simulink model "three_phase_inverter_LCL"  (R2024a)
settings: Solver=VariableStepAuto  StartTime=0.0  StopTime=10.0  RelTol=1e-3
libraries: spsSeriesRLCBranchLib x12, simulink x7, spsIGBTLib x6, slpidlib x4, spsabctodq0Lib x3, spsGroundLib x2, spsSawtoothGeneratorLib x2, spsTHDLib x2, spsDCVoltageSourceLib x1, spsThreePhaseParallelRLCBranchLib x1, spsThreePhaseVIMeasurementLib x1, sps_lib x1
settings Model: Creator=rizzilouise  LastModifiedBy=rizzilouise
settings SolverCC: ZeroCrossAlgorithm=Adaptive
settings DebuggingCC: MaskedZcDiagnostic=none  IgnoredZcDiagnostic=none  InitInArrayFormatMsg=none

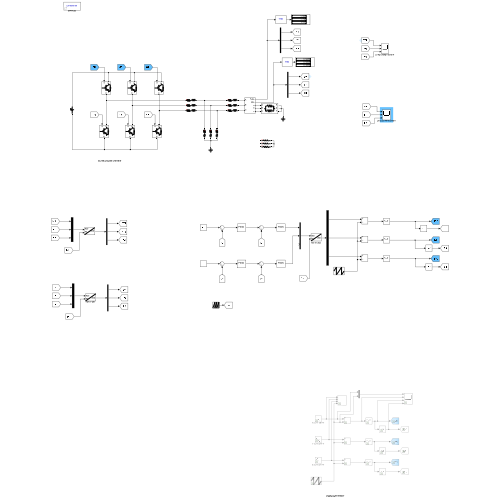
[thumbnail: Simulink's stored preview of the top-level diagram]
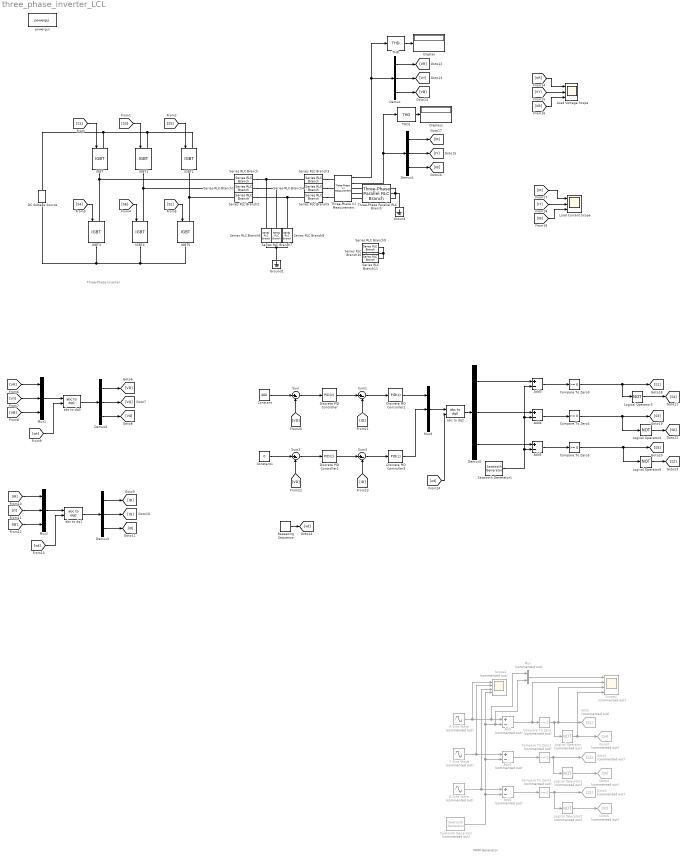
== system three_phase_inverter_LCL ==
  note: PWM Generator
  note: Three-Phase Inverter
  Add : Sum  Commented=on  Inputs=+-
  Add1 : Sum  Commented=on  Inputs=+-
  Add2 : Sum  Commented=on  Inputs=+-
  Add3 : Sum  Inputs=+-
  Add4 : Sum  Inputs=+-
  Add5 : Sum  Inputs=+-
  B Sine Wave : Sin  Commented=on  Frequency=2*pi*50  Phase=-2*pi/3  SampleTime=0
  Compare To Zero : simulink/Logic and Bit Operations/Compare To Zero  Commented=on  relop=>=  OutDataTypeStr=boolean
  Compare To Zero1 : simulink/Logic and Bit Operations/Compare To Zero  Commented=on  relop=>=  OutDataTypeStr=boolean
  Compare To Zero2 : simulink/Logic and Bit Operations/Compare To Zero  Commented=on  relop=>=  OutDataTypeStr=boolean
  Compare To Zero3 : simulink/Logic and Bit Operations/Compare To Zero  relop=>=  OutDataTypeStr=boolean
  Compare To Zero4 : simulink/Logic and Bit Operations/Compare To Zero  relop=>=  OutDataTypeStr=boolean
  Compare To Zero5 : simulink/Logic and Bit Operations/Compare To Zero  relop=>=  OutDataTypeStr=boolean
  Constant : Constant  Value=400
  Constant1 : Constant  Value=0
  DC Voltage Source : spsDCVoltageSourceLib/DC Voltage Source  Amplitude=230  Measurements=None
  Demux{,1..4} (5 alike) : Demux  Outputs=3
  Discrete PID Controller{,1..3} (4 alike) : slpidlib/PID Controller  Controller=PID  Form=Parallel  TimeDomain=Discrete-time  UseExternalTs=off  SampleTime=-1  IntegratorMethod=Forward Euler  FilterMethod=Forward Euler  ControllerParametersSource=internal  P=1  I=1  UseKiTs=off  D=0  UseExternalDerivativeSource=off  N=100  UseFilter=on  TunerSelectOption=Transfer Function Based (PID Tuner App)  InitialConditionSource=internal  InitialConditionForIntegrator=0  InitialConditionForFilter=0  DifferentiatorICPrevScaledInput=0  ExternalReset=none  TrackingMode=off  Kt=1  LimitOutput=off  SatLimitsSource=internal  UpperSaturationLimit=inf  LowerSaturationLimit=-inf  LinearizeAsGain=off  AntiWindupMode=none  Kb=1  LimitIntegrator=off  UpperIntegratorSaturationLimit=inf  LowerIntegratorSaturationLimit=-inf  POutMin=[]  POutMax=[]  IOutMin=[]  IOutMax=[]  DOutMin=[]  DOutMax=[]  NOutMin=[]  NOutMax=[]  SumOutMin=[]  SumOutMax=[]  SaturationOutMin=[]  SaturationOutMax=[]  PParamMin=[]  PParamMax=[]  IParamMin=[]  IParamMax=[]  DParamMin=[]  DParamMax=[]  NParamMin=[]  NParamMax=[]  KbParamMin=[]  KbParamMax=[]  KtParamMin=[]  KtParamMax=[]  KbOutMin=[]  KbOutMax=[]  KtOutMin=[]  KtOutMax=[]  IntegratorOutMin=[]  IntegratorOutMax=[]  FilterOutMin=[]  FilterOutMax=[]  SumI1OutMin=[]  SumI1OutMax=[]  SumI2OutMin=[]  SumI2OutMax=[]  SumI3OutMin=[]  SumI3OutMax=[]  SumI4OutMin=[]  SumI4OutMax=[]  SumDOutMin=[]  SumDOutMax=[]  DifferentiatorOutMin=[]  DifferentiatorOutMax=[]  FilterDiffOutCoefMin=[]  FilterDiffOutCoefMax=[]  ReciprocalOutMin=[]  ReciprocalOutMax=[]  SumDenOutMin=[]  SumDenOutMax=[]  SumNumOutMin=[]  SumNumOutMax=[]  DivideOutMin=[]  DivideOutMax=[]  UdiffTsProdOutMin=[]  UdiffTsProdOutMax=[]  NTsProdOutMin=[]  NTsProdOutMax=[]  UintegralTsProdOutMin=[]  UintegralTsProdOutMax=[]  UngainTsProdOutMin=[]  UngainTsProdOutMax=[]  ClampingZeroOutDataTypeStr=Inherit: Inherit via back propagation  ClampingZeroOutMin=[]  ClampingZeroOutMax=[]  FilterDenConstantOutDataTypeStr=Inherit: Inherit via back propagation  FilterDenConstantOutMin=[]  FilterDenConstantOutMax=[]  PCopyOutDataTypeStr=Inherit: Inherit via back propagation  PCopyOutMin=[]  PCopyOutMax=[]  NCopyOutDataTypeStr=Inherit: Inherit via back propagation  NCopyOutMin=[]  NCopyOutMax=[]  IntegratorContinuousStateAttributes=''  IntegratorStateMustResolveToSignalObject=off  IntegratorRTWStateStorageClass=Auto  FilterContinuousStateAttributes=''  FilterStateMustResolveToSignalObject=off  FilterRTWStateStorageClass=Auto  ParallelPVariant=InternalParameters  IdealPVariant=Disabled  IVariant=InternalParameters  DVariant=InternalParameters  IntegratorVariant=Discrete  SatVariant=Disabled  AWVariant=Passthrough  PCopyVariant=Disabled  TRVariant=Disabled  FdbkBlocksVariant=Forward  IdealPFdbkVariant=Disabled  SatFdbkVariant=Disabled  DerivativeFilterVariant=ForwardEulerFilter  NVariant=InternalParameters  NCopyVariant=Disabled  FilterICVariant=InternalICsFilter  IntegratorICVariant=InternalICs  ExternalResetVariant=Disabled  TRSumVariant=Passthrough  SumFdbkVariant=Disabled  SumVariant=Sum_PID  TsampFilterVariant=InternalTs  TsampNgainVariant=Passthrough  TsampIntegralVariant=Disabled_SignalSpec  ExternalSaturationOutDataTypeStr=Inherit: Same as second input  DerivativeSourceVariant=ErrorSignal
      settings: LibrarySourceBlock=simulink/Discrete/Discrete PID Controller
  Display : Display
  Display1 : Display
  Goto : Goto  Commented=on  GotoTag=S1
  Goto1 : Goto  Commented=on  GotoTag=S3
  Goto2 : Goto  Commented=on  GotoTag=S5
  Goto3 : Goto  Commented=on  GotoTag=S4
  Goto4 : Goto  Commented=on  GotoTag=S6
  Goto5 : Goto  Commented=on  GotoTag=S2
  Ground : spsGroundLib/Ground  LConnTagsString=a
  Ground1 : spsGroundLib/Ground  LConnTagsString=a
  IGBT{,1..5} (6 alike) : spsIGBTLib/IGBT  Ron=0.001  Lon=0  Vf=1  Tf=1e-6  Tt=2e-6  IC=0  Rs=1e5  Cs=inf  Measurements=off
  Load Current Scope : Scope  NumInputPorts=3
  Load Voltage Scope : Scope  NumInputPorts=3
  Logical Operator : Logic  Commented=on  Operator=NOT  AllPortsSameDT=off  OutDataTypeStr=boolean
  Logical Operator1 : Logic  Commented=on  Operator=NOT  AllPortsSameDT=off  OutDataTypeStr=boolean
  Logical Operator2 : Logic  Commented=on  Operator=NOT  AllPortsSameDT=off  OutDataTypeStr=boolean
  Logical Operator3 : Logic  Operator=NOT  AllPortsSameDT=off  OutDataTypeStr=boolean
  Logical Operator4 : Logic  Operator=NOT  AllPortsSameDT=off  OutDataTypeStr=boolean
  Logical Operator5 : Logic  Operator=NOT  AllPortsSameDT=off  OutDataTypeStr=boolean
  Mux : Mux  Commented=on  Inputs=2
  Mux1 : Mux  Inputs=3
  Mux2 : Mux  Inputs=3
  Mux3 : Mux  Inputs=3
  R Sine Wave : Sin  Commented=on  Frequency=2*pi*50  SampleTime=0
  Repeating Sequence : simulink/Sources/Repeating Sequence  rep_seq_t=[0 20e-3]  rep_seq_y=[0 2*pi]
  Sawtooth Generator : spsSawtoothGeneratorLib/Sawtooth Generator  Commented=on  Freq=10e3  Phase=180  Ts=0
  Sawtooth Generator1 : spsSawtoothGeneratorLib/Sawtooth Generator  Freq=10e3  Phase=180  Ts=0
  Scope1 : Scope  Commented=on  NumInputPorts=4
  Scope2 : Scope  Commented=on  NumInputPorts=4
  Series RLC Branch{,1..5} (6 alike) : spsSeriesRLCBranchLib/Series RLC Branch  LConnTagsString=__new0  RConnTagsString=__new0  BranchType=RL  Resistance=20e-3  Inductance=500e-6  SetiL0=off  InitialCurrent=0  Capacitance=1e-6  Setx0=off  InitialVoltage=0  Measurements=None
  Series RLC Branch10 : spsSeriesRLCBranchLib/Series RLC Branch  LConnTagsString=__new0  RConnTagsString=__new0  BranchType=R  Resistance=1.1  Inductance=1e-3  SetiL0=off  InitialCurrent=0  Capacitance=1e-6  Setx0=off  InitialVoltage=0  Measurements=None
  Series RLC Branch11 : spsSeriesRLCBranchLib/Series RLC Branch  LConnTagsString=__new0  RConnTagsString=__new0  BranchType=R  Resistance=1.1  Inductance=1e-3  SetiL0=off  InitialCurrent=0  Capacitance=1e-6  Setx0=off  InitialVoltage=0  Measurements=None
  Series RLC Branch6 : spsSeriesRLCBranchLib/Series RLC Branch  LConnTagsString=__new0  RConnTagsString=__new0  BranchType=RC  Resistance=20e-3  Inductance=1e-3  SetiL0=off  InitialCurrent=0  Capacitance=100e-6  Setx0=off  InitialVoltage=0  Measurements=None
  Series RLC Branch7 : spsSeriesRLCBranchLib/Series RLC Branch  LConnTagsString=__new0  RConnTagsString=__new0  BranchType=RC  Resistance=20e-3  Inductance=1e-3  SetiL0=off  InitialCurrent=0  Capacitance=100e-6  Setx0=off  InitialVoltage=0  Measurements=None
  Series RLC Branch8 : spsSeriesRLCBranchLib/Series RLC Branch  LConnTagsString=__new0  RConnTagsString=__new0  BranchType=RC  Resistance=20e-3  Inductance=1e-3  SetiL0=off  InitialCurrent=0  Capacitance=100e-6  Setx0=off  InitialVoltage=0  Measurements=None
  Series RLC Branch9 : spsSeriesRLCBranchLib/Series RLC Branch  LConnTagsString=__new0  RConnTagsString=__new0  BranchType=R  Resistance=1.1  Inductance=1e-3  SetiL0=off  InitialCurrent=0  Capacitance=1e-6  Setx0=off  InitialVoltage=0  Measurements=None
  Sum{,1..3} (4 alike) : Sum  Inputs=|+-
  THD : spsTHDLib/THD  Freq=60  Ts=0
  THD1 : spsTHDLib/THD  Freq=60  Ts=0
  Three-Phase Parallel RLC Branch : spsThreePhaseParallelRLCBranchLib/Three-Phase Parallel RLC Branch  LConnTagsString=A|B|C  RConnTagsString=A|B|C  BranchType=RL  Resistance=10  Inductance=2.5e-3  Capacitance=1e-6  Measurements=None
  Three-Phase V-I Measurement : spsThreePhaseVIMeasurementLib/Three-Phase V-I Measurement  VoltageMeasurement=phase-to-ground  SetLabelV=off  LabelV=Vabc  Vpu=off  VpuLL=off  CurrentMeasurement=yes  SetLabelI=off  LabelI=Iabc  Ipu=off  Pbase=100e6  Vbase=500e3  OutputType=Complex  PhasorSimulation=off  PSBequivalent=0
  Y Sine Wave : Sin  Commented=on  Frequency=2*pi*50  Phase=2*pi/3  SampleTime=0
  abc to dq0 : spsabctodq0Lib/abc to dq0  Alignment=90 degrees behind phase A axis
  abc to dq1 : spsabctodq0Lib/abc to dq0  Alignment=90 degrees behind phase A axis
  abc to dq2 : spsabctodq0Lib/abc to dq0  Alignment=90 degrees behind phase A axis
  powergui : sps_lib/powergui  Priority=1  SimulationMode=Continuous  SampleTime=50e-6  frequency=60  Iterations=50  frequencyindice=0  Pbase=100e6  ErrMax=1e-4  UnitsV=kV  UnitsW=MW  buscounter=0  FunctionMessages=off  echomessages=off  EnableUseOfTLC=off  CurrentSourceSwitches=off  DisableSnubberDevices=off  DisableRonSwitches=off  DisableVfSwitches=off  DisplayEquations=off  AutomaticDiscreteSolvers=off  SolverType=Tustin/Backward Euler (TBE)  Interpol=off  ExternalGateDelay=off  methode=off  Ts=100  x0status=blocks  SPID=on  SwTol=0  HookPort=off  NonlinearTolerance=1e-4  nMaxIteration=100  ContinueOnMaxIteration=off  RestoreLinks=warning  ResistiveCurrentMeasurement=off  Frange=[0:2:500]  Ylog=off  Xlog=on  ShowGrid=off  save=off  variable=ZData  structure=0  ZoomFFT=off  StartTime=0.0  cycles=1  DisplayStyle=1  fundamental=60  FreqAxis=off  MaxFrequency=1000  frequencyindicesteady=1  RmsSteady=1  display=off
  wires:
  Y Sine Wave/1 -> Scope1/2, Add1/1
  Compare To Zero/1 -> Logical Operator/1, Scope2/3, Goto/1
  B Sine Wave/1 -> Scope1/3, Add2/1
  Logical Operator/1 -> Goto3/1, Scope2/4
  [S1] -> IGBT/1
  Compare To Zero2/1 -> Logical Operator2/1, Goto2/1
  Logical Operator1/1 -> Goto4/1
  Logical Operator2/1 -> Goto5/1
  Sawtooth Generator/1 -> Add2/2, Add1/2, Scope1/4, Mux/2, Add/2
  R Sine Wave/1 -> Mux/1, Add/1, Scope1/1
  Add1/1 -> Compare To Zero1/1
  Compare To Zero1/1 -> Logical Operator1/1, Goto1/1
  [S4] -> IGBT3/1
  Add2/1 -> Compare To Zero2/1
  [S2] -> IGBT5/1
  Add/1 -> Scope2/2, Compare To Zero/1
  Three-Phase V-I Measurement/2 -> Demux1/1, THD1/1
  [S3] -> IGBT1/1
  [S6] -> IGBT4/1
  THD1/1 -> Display1/1
  Mux/1 -> Scope2/1
  Three-Phase V-I Measurement/1 -> THD/1, Demux/1
  [S5] -> IGBT2/1
  THD/1 -> Display/1
  [VY] -> Mux1/2
  [VR] -> Mux1/1
  [VB] -> Mux1/3
  Mux1/1 -> abc to dq0/1
  abc to dq0/1 -> Demux2/1
  Demux2/2 -> [VQ]
  Demux2/1 -> [VD]
  Demux2/3 -> [V0]
  [wt] -> abc to dq0/2
  abc to dq1/1 -> Demux3/1
  [IY] -> Mux2/2
  [IB] -> Mux2/3
  Demux3/2 -> [IQ]
  Demux3/1 -> [ID]
  [IR] -> Mux2/1
  [wt] -> abc to dq1/2
  Demux3/3 -> [I0]
  Mux2/1 -> abc to dq1/1
  [VR] -> Load Voltage Scope/1
  [VY] -> Load Voltage Scope/2
  [VB] -> Load Voltage Scope/3
  Demux/2 -> [VY]
  Demux/3 -> [VB]
  Demux/1 -> [VR]
  [IY] -> Load Current Scope/2
  [IR] -> Load Current Scope/1
  [IB] -> Load Current Scope/3
  Demux1/1 -> [IR]
  Demux1/2 -> [IY]
  Demux1/3 -> [IB]
  Constant/1 -> Sum/1
  [VD] -> Sum/2
  Sum/1 -> Discrete PID Controller/1
  Discrete PID Controller/1 -> Sum1/1
  [ID] -> Sum1/2
  Sum1/1 -> Discrete PID Controller1/1
  Constant1/1 -> Sum2/1
  [ID] -> Sum3/2
  [VD] -> Sum2/2
  Discrete PID Controller2/1 -> Sum3/1
  Sum3/1 -> Discrete PID Controller3/1
  Sum2/1 -> Discrete PID Controller2/1
  Discrete PID Controller1/1 -> Mux3/1
  Discrete PID Controller3/1 -> Mux3/2
  Mux3/1 -> abc to dq2/1
  [wt] -> abc to dq2/2
  abc to dq2/1 -> Demux4/1
  Compare To Zero3/1 -> Logical Operator3/1, [S1]
  Logical Operator3/1 -> [S4]
  Demux4/1 -> Add3/1
  Compare To Zero5/1 -> [S5], Logical Operator5/1
  Compare To Zero4/1 -> [S3], Logical Operator4/1
  Add4/1 -> Compare To Zero4/1
  Add3/1 -> Compare To Zero3/1
  Add5/1 -> Compare To Zero5/1
  Demux4/2 -> Add4/1
  Sawtooth Generator1/1 -> Add5/2, Add4/2, Add3/2
  Demux4/3 -> Add5/1
  Logical Operator4/1 -> [S6]
  Logical Operator5/1 -> [S2]
  Repeating Sequence/1 -> [wt]
  connections:
  IGBT5/RConn1 -- IGBT3/RConn1 -- DC Voltage Source/LConn1 -- IGBT4/RConn1
  DC Voltage Source/RConn1 -- IGBT/LConn1 -- IGBT1/LConn1 -- IGBT2/LConn1
  IGBT1/RConn1 -- Series RLC Branch1/LConn1 -- IGBT4/LConn1
  IGBT2/RConn1 -- Series RLC Branch2/LConn1 -- IGBT5/LConn1
  IGBT/RConn1 -- IGBT3/LConn1 -- Series RLC Branch/LConn1
  Series RLC Branch/RConn1 -- Series RLC Branch3/LConn1 -- Series RLC Branch6/LConn1
  Series RLC Branch1/RConn1 -- Series RLC Branch7/LConn1 -- Series RLC Branch4/LConn1
  Series RLC Branch2/RConn1 -- Series RLC Branch8/LConn1 -- Series RLC Branch5/LConn1
  Series RLC Branch6/RConn1 -- Ground1/LConn1 -- Series RLC Branch8/RConn1 -- Series RLC Branch7/RConn1
  Series RLC Branch5/RConn1 -- Three-Phase V-I Measurement/LConn3
  Series RLC Branch4/RConn1 -- Three-Phase V-I Measurement/LConn2
  Series RLC Branch3/RConn1 -- Three-Phase V-I Measurement/LConn1
  Series RLC Branch9/RConn1 -- Series RLC Branch11/RConn1 -- Series RLC Branch10/RConn1
  Three-Phase Parallel RLC Branch/LConn1 -- Three-Phase V-I Measurement/RConn1
  Three-Phase Parallel RLC Branch/LConn2 -- Three-Phase V-I Measurement/RConn2
  Three-Phase Parallel RLC Branch/LConn3 -- Three-Phase V-I Measurement/RConn3
  Three-Phase Parallel RLC Branch/RConn1 -- Ground/LConn1 -- Three-Phase Parallel RLC Branch/RConn3 -- Three-Phase Parallel RLC Branch/RConn2
